simulink model "AGC30Model_ex1_11"  (R2021a)
settings: Solver=ode4  StartTime=stime  StopTime=etime  FixedStep=dtload  RelTol=1e-3
values from neighbouring files (symbols this model uses):
  AL_A = 0.3    [init_lfc_model.m]
  AL_B = 0.3    [init_lfc_model.m]
  DELTA_CC = Delta_cc_ty(TY_CC)    [load_thermal_constants.m]
  DELTA_ST = Delta_st_ty(TY_ST)    [load_thermal_constants.m]
  dtload = 0.1    [initset_dataload.m]
  F0 = 60    [init_inertia_model.m]    (also in initset_inertia.m)
  FFCS0_CC = (WF0_CC-WF_MIN_CC)./(1.0-WF_MIN_CC)    [calc_thermal_init_values.m]    (also in init_thermals.m)
  FGT_CC = Fgt_cc_ty(TY_CC)    [load_thermal_constants.m]
  FX_FB_CC = Fx_fb_cc_ty(:,TY_CC)    [load_thermal_constants.m]
  FX_FB_ST = Fx_fb_st_ty(:,TY_ST)    [load_thermal_constants.m]
  FX_FB_WT = FX_FB_WT_ty(:,TY_WT)    [load_const_hydro_constants.m]
  FX_N_GN_VA = FX_N_GN_VA_ty(:,TY_VA)    [load_var_hydro_constants.m]
  FX_N_PM_VA = FX_N_PM_VA_ty(:,TY_VA)    [load_var_hydro_constants.m]
  FX_PTHD_ST = Fx_pthd_st_ty(:,TY_ST)    [load_thermal_constants.m]
  FX_T_PM_VA = FX_T_PM_VA_ty(:,TY_VA)    [load_var_hydro_constants.m]
  FX_TE1_CC = Fx_te1_cc_ty(:,TY_CC)    [load_thermal_constants.m]
  FX_TE2_CC = Fx_te2_cc_ty(:,TY_CC)    [load_thermal_constants.m]
  FX_Y_GN_VA = FX_Y_GN_VA_ty(:,TY_VA)    [load_var_hydro_constants.m]
  FX_Y_PM_VA = FX_Y_PM_VA_ty(:,TY_VA)    [load_var_hydro_constants.m]
  FY_FB_CC = Fy_fb_cc_ty(:,TY_CC)    [load_thermal_constants.m]
  FY_FB_ST = Fy_fb_st_ty(:,TY_ST)    [load_thermal_constants.m]
  FY_FB_WT = FY_FB_WT_ty(:,TY_WT)    [load_const_hydro_constants.m]
  FY_N_GN_VA = FY_N_GN_VA_ty(:,TY_VA)    [load_var_hydro_constants.m]
  FY_N_PM_VA = FY_N_PM_VA_ty(:,TY_VA)    [load_var_hydro_constants.m]
  FY_PTHD_ST = Fy_pthd_st_ty(:,TY_ST)    [load_thermal_constants.m]
  FY_T_PM_VA = FY_T_PM_VA_ty(:,TY_VA)    [load_var_hydro_constants.m]
  FY_TE1_CC = Fy_te1_cc_ty(:,TY_CC)    [load_thermal_constants.m]
  FY_TE2_CC = Fy_te2_cc_ty(:,TY_CC)    [load_thermal_constants.m]
  FY_Y_GN_VA = FY_Y_GN_VA_ty(:,TY_VA)    [load_var_hydro_constants.m]
  FY_Y_PM_VA = FY_Y_PM_VA_ty(:,TY_VA)    [load_var_hydro_constants.m]
  G_cost = [Cost(:,3) ... (first row only)    [initset_dataload.m]
  G_down_limit = max(G_down_limit, G_out_pre - G_speed*5)    [calc_edc_output.m]    (also in edc.m; initset_dataload.m = csvread('G_down_plan_limit.csv',0,1))
  G_G_ST = G_g_st_ty(TY_ST)    [load_thermal_constants.m]
  G_speed = u(220:249,1)    [calc_edc_output.m]    (also in edc.m; initset_dataload.m = G_speed(:,1))
  GF_CC = [1, 1, 1, 1, 1,            1, 1, 1, 1, 1]    [init_thermal_model.m]
  GF_ST = [1, 1, 1, 1, 1, 1, 1,            1, 1, 1, 1,            1, 1, 1, 1, 1, 1]    [init_thermal_model.m]
  GMW_CC = Gmw_cc_ty(TY_CC)    [load_thermal_constants.m]
  GMW_ST = Gmw_st_ty(TY_ST)    [load_thermal_constants.m]
  GMW_VA = GMW_VA_ty(TY_VA)    [load_var_hydro_constants.m]
  GMW_WT = GMW_WT_ty(TY_WT)    [load_const_hydro_constants.m]
  HC_CC = Hc_cc_ty(TY_CC)    [load_thermal_constants.m]
  HT_CC = Ht_cc_ty(TY_CC)    [load_thermal_constants.m]
  IGV0_CC = WF0_CC    [calc_thermal_init_values.m]    (also in init_thermals.m)
  inertia_input = inertia_input'    [initset_dataload.m]
  K1_CONV_VA = K1_CONV_VA_ty(TY_VA)    [load_var_hydro_constants.m]
  K1_CONV_WT = K1_CONV_WT_ty(TY_WT)    [load_const_hydro_constants.m]
  K2_SERV_VA = K2_SERV_VA_ty(TY_VA)    [load_var_hydro_constants.m]
  K2_SERV_WT = K2_SERV_WT_ty(TY_WT)    [load_const_hydro_constants.m]
  K_A = 0.1    [init_lfc_model.m]
  K_B = 0.1    [init_lfc_model.m]
  K_G_ST = K_g_st_ty(TY_ST)    [load_thermal_constants.m]
  K_IGV_CC = K_igv_cc_ty(TY_CC)    [load_thermal_constants.m]
  K_L = 2.0    (= 2)    [init_inertia_model.m]    (also in initset_inertia.m)
  K_MW_GV_VA = K_MW_GV_VA_ty(TY_VA)    [load_var_hydro_constants.m]
  K_PREF_ST = K_pref_st_ty(TY_ST)    [load_thermal_constants.m]
  K_SD_VA = K_SD_VA_ty(TY_VA)    [load_var_hydro_constants.m]
  K_SD_WT = K_SD_WT_ty(TY_WT)    [load_const_hydro_constants.m]
  K_SEQ_WT = K_SEQ_WT_ty(TY_WT)    [load_const_hydro_constants.m]
  K_TE_CC = K_te_cc_ty(TY_CC)    [load_thermal_constants.m]
  KD_PID_VA = KD_PID_VA_ty(TY_VA)    [load_var_hydro_constants.m]
  KD_PID_WT = KD_PID_WT_ty(TY_WT)    [load_const_hydro_constants.m]
  KD_SG_GN_VA = KD_SG_GN_VA_ty(TY_VA)    [load_var_hydro_constants.m]
  KD_SG_PM_VA = KD_SG_PM_VA_ty(TY_VA)    [load_var_hydro_constants.m]
  KGT_CC = FGT_CC./((TFR_CC-TER_CC)-(TDR_CC-TIR_CC))    [calc_thermal_init_values.m]    (also in init_thermals.m)
  KI_PID_VA = KI_PID_VA_ty(TY_VA)    [load_var_hydro_constants.m]
  KI_PID_WT = KI_PID_WT_ty(TY_WT)    [load_const_hydro_constants.m]
  KI_SG_GN_VA = KI_SG_GN_VA_ty(TY_VA)    [load_var_hydro_constants.m]
  KI_SG_PM_VA = KI_SG_PM_VA_ty(TY_VA)    [load_var_hydro_constants.m]
  KP_A = 1.0    (= 1)    [init_lfc_model.m]
  KP_B = 1.0    (= 1)    [init_lfc_model.m]
  KP_PID_VA = KP_PID_VA_ty(TY_VA)    [load_var_hydro_constants.m]
  KP_PID_WT = KP_PID_WT_ty(TY_WT)    [load_const_hydro_constants.m]
  KP_SG_GN_VA = KP_SG_GN_VA_ty(TY_VA)    [load_var_hydro_constants.m]
  KP_SG_PM_VA = KP_SG_PM_VA_ty(TY_VA)    [load_var_hydro_constants.m]
  KST_CC = (1.0-FGT_CC)./TER_CC    [calc_thermal_init_values.m]    (also in init_thermals.m)
  L_FUEL_CC = L_fuel_cc_ty(TY_CC)    [load_thermal_constants.m]
  L_G_ST = L_g_st_ty(TY_ST)    [load_thermal_constants.m]
  L_IGV_CC = L_igv_cc_ty(TY_CC)    [load_thermal_constants.m]
  L_LL_ST = L_ll_st_ty(TY_ST)    [load_thermal_constants.m]
  L_MWD_CC = L_mwd_cc_ty(TY_CC)    [load_thermal_constants.m]
  L_MWD_GN_VA = L_MWD_GN_VA_ty(TY_VA)    [load_var_hydro_constants.m]
  L_MWD_PM_VA = L_MWD_PM_VA_ty(TY_VA)    [load_var_hydro_constants.m]
  L_MWD_ST = L_mwd_st_ty(TY_ST)    [load_thermal_constants.m]
  L_MWD_WT = L_MWD_WT_ty(TY_WT)    [load_const_hydro_constants.m]
  L_PREF_CC = L_pref_cc_ty(TY_CC)    [load_thermal_constants.m]
  L_PREF_ST = L_pref_st_ty(TY_ST)    [load_thermal_constants.m]
  LFC_cycle = 5.0    (= 5)    [init_lfc_model.m]
  load_input = load_input(:,stime+1:etime+1)    [initset_dataload.m]
  M_VA = M_VA_ty(TY_VA)    [load_var_hydro_constants.m]
  MVABase = 1000    [init_inertia_model.m]    (also in initset_inertia.m)
  MW0_ST = zeros(1,17)    [calc_thermal_init_values.m]    (also in init_thermals.m)
  MW0_WT = zeros(1,2)    [calc_const_hydro_init_values.m]    (also in init_conhydros.m)
  P_G_CONV_WT = P_G_CONV_WT_ty(TY_WT)    [load_const_hydro_constants.m]
  PG_INIT_CC = PMWD_SCHEDULE(1,19:28)'    [calc_thermal_init_values.m]    (also in init_thermals.m)
  PLM_CC = Plm_cc_ty(TY_CC)    [load_thermal_constants.m]
  PLM_ST = Plm_st_ty(TY_ST)    [load_thermal_constants.m]
  PMAX_B = 360.0    (= 360)    [init_lfc_model.m]
  PMIN_B = -360.0    (= -360)    [init_lfc_model.m]
  PMST0_CC = zeros(1, 10)    [calc_thermal_init_values.m]    (also in init_thermals.m)
  PMWD_EDC0 = zeros(1,30)    [init_edc_model.m]    (also in initset_edc.m)
  PMWD_SCHEDULE = u(3:32,1)    [calc_edc_output.m]    (also in edc.m; init_edc_model.m = g_out_input'; initset_edc.m = g_out_input')
  PRC_CC = Prc_cc_ty(TY_CC)    [load_thermal_constants.m]
  PRT_CC = PRC_CC.*(1-EP_CC)    [calc_thermal_init_values.m]    (also in init_thermals.m)
  PTH0_ST = zeros(1,17)    [calc_thermal_init_values.m]    (also in init_thermals.m)
  R_LL_ST = R_ll_st_ty(TY_ST)    [load_thermal_constants.m]
  R_MWD_CC = R_mwd_cc_ty(TY_CC)    [load_thermal_constants.m]
  R_MWD_ST = R_mwd_st_ty(TY_ST)    [load_thermal_constants.m]
  R_PREF_CC = R_pref_cc_ty(TY_CC)    [load_thermal_constants.m]
  RA_A = G_speed'    [init_lfc_model.m]
  RA_B = 96.0    (= 96)    [init_lfc_model.m]
  RATE_GN_VA = RATE_GN_VA_ty(TY_VA)    [load_var_hydro_constants.m]
  RATE_PM_VA = RATE_PM_VA_ty(TY_VA)    [load_var_hydro_constants.m]
  RC_CC = Rc_cc_ty(TY_CC)    [load_thermal_constants.m]
  RT_CC = Rt_cc_ty(TY_CC)    [load_thermal_constants.m]
  SW_T_ST = Sw_t_st_ty(TY_ST)    [load_thermal_constants.m]
  T1_B_ST = T1_b_st_ty(TY_ST)    [load_thermal_constants.m]
  T1_CONV_VA = T1_CONV_VA_ty(TY_VA)    [load_var_hydro_constants.m]
  T1_CONV_WT = T1_CONV_WT_ty(TY_WT)    [load_const_hydro_constants.m]
  T1_G_ST = T1_g_st_ty(TY_ST)    [load_thermal_constants.m]
  T2_B_ST = T2_b_st_ty(TY_ST)    [load_thermal_constants.m]
  ... (+53 more)
undefined symbols (not defined in the file or in its folder): DELTA_B, DiscIntNeverNeededParam, FX_FB_ST_OA, FX_PTHD_ST_OA, FY_FB_ST_OA, FY_PTHD_ST_OA, G_G_ST_OA, K_G_ST_OA, K_PREF_ST_OA, MW0_ST_OA, N_GN_INIT_VA, N_PM_INIT_VA, PLM_B, R_LL_ST_OA, T1_B_ST_OA, T1_G_ST_OA, T2_B_ST_OA, T2_G_ST_OA, T3_B_ST_OA, T4_G_ST_OA, T5_G_ST_OA, T_LL_ST_OA, T_PREF_ST_OA, Y_GN_INIT_VA, Y_PM_INIT_VA
libraries: simulink_extras x87, simulink x42, pid_lib x1
(part 4 of 5)

== system AGC30Model_ex1_11/可変速揚水発電機/可変速揚水/連続出力切替 ==
  モデル : Inport
  運転モード : Inport  Port=2
  MWD : Inport  Port=3
  Add : Sum
  Constant : Constant  Value=0
  Gain : Gain  Gain=-1
  Gain1 : Gain  Gain=-1
  Gain2 : Gain  Gain=-1
  MWD使用時に レートを制限 : Switch  Threshold=1
  MWD使用時はMWD-モデル モデル使用時は0 : Switch  Threshold=1
  MWD使用時はMWD-モデルに追従 モデル使用時はレートでMWD-モデルから0へ変化 （MWD⇒モデル時に不連続打消し分として使用） : simulink/Discontinuities/Rate Limiter Dynamic
  Scope1 : Scope
  Scope2 : Scope
  Subtract : Sum  Inputs=-+
  Switch1 : Switch  Threshold=1
  ∞ : Constant  Value=9999
  モデル使用時に レートを制限 : Switch  Threshold=1
  モデル使用時はモデル-MWD MWD使用時は0 : Switch  Threshold=1
  モデル使用時はモデル-MWDに追従 MWD使用時はレートでモデル-MWDから0に変化 （モデル⇒MWD時に不連続打消し分として使用） : simulink/Discontinuities/Rate Limiter Dynamic
  不連続 打消し分 : Switch  Threshold=1
  不連続分を戻すレート : Constant  Value=0.0001
  出力 : Outport  VectorParamsAs1DForOutWhenUnconnected=off
  wires:
  MWD/1 -> Subtract/2, Switch1/3
  モデル/1 -> Switch1/1, Subtract/1
  Constant/1 -> MWD使用時はMWD-モデル モデル使用時は0/1, モデル使用時はモデル-MWD MWD使用時は0/3
  Subtract/1 -> Gain2/1, MWD使用時はMWD-モデル モデル使用時は0/3
  MWD使用時はMWD-モデル モデル使用時は0/1 -> MWD使用時はMWD-モデルに追従 モデル使用時はレートでMWD-モデルから0へ変化 （MWD⇒モデル時に不連続打消し分として使用）/2
  モデル使用時はモデル-MWD MWD使用時は0/1 -> モデル使用時はモデル-MWDに追従 MWD使用時はレートでモデル-MWDから0に変化 （モデル⇒MWD時に不連続打消し分として使用）/2
  モデル使用時はモデル-MWDに追従 MWD使用時はレートでモデル-MWDから0に変化 （モデル⇒MWD時に不連続打消し分として使用）/1 -> 不連続 打消し分/3
  MWD使用時はMWD-モデルに追従 モデル使用時はレートでMWD-モデルから0へ変化 （MWD⇒モデル時に不連続打消し分として使用）/1 -> 不連続 打消し分/1
  Add/1 -> 出力/1
  不連続分を戻すレート/1 -> モデル使用時に レートを制限/1, MWD使用時に レートを制限/3
  ∞/1 -> モデル使用時に レートを制限/3, MWD使用時に レートを制限/1
  モデル使用時に レートを制限/1 -> MWD使用時はMWD-モデルに追従 モデル使用時はレートでMWD-モデルから0へ変化 （MWD⇒モデル時に不連続打消し分として使用）/1, Gain/1
  MWD使用時に レートを制限/1 -> モデル使用時はモデル-MWDに追従 MWD使用時はレートでモデル-MWDから0に変化 （モデル⇒MWD時に不連続打消し分として使用）/1, Gain1/1
  Gain/1 -> MWD使用時はMWD-モデルに追従 モデル使用時はレートでMWD-モデルから0へ変化 （MWD⇒モデル時に不連続打消し分として使用）/3
  Gain1/1 -> モデル使用時はモデル-MWDに追従 MWD使用時はレートでモデル-MWDから0に変化 （モデル⇒MWD時に不連続打消し分として使用）/3
  Gain2/1 -> モデル使用時はモデル-MWD MWD使用時は0/1
  Switch1/1 -> Scope2/1, Add/1
  不連続 打消し分/1 -> Add/2, Scope1/1
  運転モード/1 -> Switch1/2, MWD使用時はMWD-モデル モデル使用時は0/2, モデル使用時はモデル-MWD MWD使用時は0/2, モデル使用時に レートを制限/2, MWD使用時に レートを制限/2, 不連続 打消し分/2

== system AGC30Model_ex1_11/定速揚水発電プラント/Water1/U=1.2L=1 ==
  Inport : Inport
  Constant : Constant  Value=upper_limit
  Constant1 : Constant  Value=lower_limit
  Constant2 : Constant  Value=0
  Constant3 : Constant  Value=0
  Constant4 : Constant  Value=0
  Integrator : Integrator  InitialCondition=X0
  Logical Operator : Logic
  Logical Operator1 : Logic  Operator=OR
  Logical Operator2 : Logic  Operator=OR
  Relational operator : RelationalOperator  Operator=<=  RndMeth=Nearest  InputSameDT=on
  Relational operator1 : RelationalOperator  RndMeth=Nearest  InputSameDT=on
  Relational operator2 : RelationalOperator  Operator=<=  RndMeth=Nearest  InputSameDT=on
  Relational operator3 : RelationalOperator  RndMeth=Nearest  InputSameDT=on
  Saturation : Saturate  UpperLimit=upper_limit  LowerLimit=lower_limit
  Switch : Switch  Threshold=0.5  SaturateOnIntegerOverflow=on  InputSameDT=on
  Outport : Outport  InitialOutput=0  VectorParamsAs1DForOutWhenUnconnected=off
  wires:
  Saturation/1 -> Outport/1
  Inport/1 -> Switch/1, Relational operator2/1, Relational operator3/1
  Switch/1 -> Integrator/1
  Constant/1 -> Relational operator/2
  Constant1/1 -> Relational operator1/2
  Logical Operator/1 -> Switch/2
  Constant2/1 -> Switch/3
  Relational operator/1 -> Logical Operator1/1
  Relational operator2/1 -> Logical Operator1/2
  Logical Operator1/1 -> Logical Operator/1
  Relational operator1/1 -> Logical Operator2/1
  Relational operator3/1 -> Logical Operator2/2
  Logical Operator2/1 -> Logical Operator/2
  Constant3/1 -> Relational operator2/2
  Constant4/1 -> Relational operator3/2
  Integrator/1 -> Saturation/1, Relational operator1/1, Relational operator/1

== system AGC30Model_ex1_11/定速揚水発電プラント/Water1/U=1L=0 ==
  Inport : Inport
  Constant : Constant  Value=upper_limit
  Constant1 : Constant  Value=lower_limit
  Constant2 : Constant  Value=0
  Constant3 : Constant  Value=0
  Constant4 : Constant  Value=0
  Integrator : Integrator  InitialCondition=X0
  Logical Operator : Logic
  Logical Operator1 : Logic  Operator=OR
  Logical Operator2 : Logic  Operator=OR
  Relational operator : RelationalOperator  Operator=<=  RndMeth=Nearest  InputSameDT=on
  Relational operator1 : RelationalOperator  RndMeth=Nearest  InputSameDT=on
  Relational operator2 : RelationalOperator  Operator=<=  RndMeth=Nearest  InputSameDT=on
  Relational operator3 : RelationalOperator  RndMeth=Nearest  InputSameDT=on
  Saturation : Saturate  UpperLimit=upper_limit  LowerLimit=lower_limit
  Switch : Switch  Threshold=0.5  SaturateOnIntegerOverflow=on  InputSameDT=on
  Outport : Outport  InitialOutput=0  VectorParamsAs1DForOutWhenUnconnected=off
  wires:
  Constant4/1 -> Relational operator3/2
  Constant3/1 -> Relational operator2/2
  Logical Operator2/1 -> Logical Operator/2
  Relational operator3/1 -> Logical Operator2/2
  Relational operator1/1 -> Logical Operator2/1
  Logical Operator1/1 -> Logical Operator/1
  Relational operator2/1 -> Logical Operator1/2
  Relational operator/1 -> Logical Operator1/1
  Constant2/1 -> Switch/3
  Logical Operator/1 -> Switch/2
  Constant1/1 -> Relational operator1/2
  Constant/1 -> Relational operator/2
  Switch/1 -> Integrator/1
  Inport/1 -> Switch/1, Relational operator2/1, Relational operator3/1
  Integrator/1 -> Relational operator1/1, Relational operator/1, Saturation/1
  Saturation/1 -> Outport/1

== system AGC30Model_ex1_11/定速揚水発電プラント/Water1/連続出力切替 ==
  モデル : Inport
  運転モード : Inport  Port=2
  MWD : Inport  Port=3
  Add : Sum
  Constant : Constant  Value=0
  Gain : Gain  Gain=-1
  Gain1 : Gain  Gain=-1
  Gain2 : Gain  Gain=-1
  MWD使用時に レートを制限 : Switch  Threshold=1
  MWD使用時はMWD-モデル モデル使用時は0 : Switch  Threshold=1
  MWD使用時はMWD-モデルに追従 モデル使用時はレートでMWD-モデルから0へ変化 （MWD⇒モデル時に不連続打消し分として使用） : simulink/Discontinuities/Rate Limiter Dynamic
  Subtract : Sum  Inputs=-+
  Switch1 : Switch  Threshold=1
  ∞ : Constant  Value=9999
  モデル使用時に レートを制限 : Switch  Threshold=1
  モデル使用時はモデル-MWD MWD使用時は0 : Switch  Threshold=1
  モデル使用時はモデル-MWDに追従 MWD使用時はレートでモデル-MWDから0に変化 （モデル⇒MWD時に不連続打消し分として使用） : simulink/Discontinuities/Rate Limiter Dynamic
  不連続 打消し分 : Switch  Threshold=1
  不連続分を戻すレート : Constant  Value=0.0001
  出力 : Outport  VectorParamsAs1DForOutWhenUnconnected=off
  wires:
  MWD/1 -> Subtract/2, Switch1/3
  モデル/1 -> Switch1/1, Subtract/1
  Constant/1 -> MWD使用時はMWD-モデル モデル使用時は0/1, モデル使用時はモデル-MWD MWD使用時は0/3
  Subtract/1 -> Gain2/1, MWD使用時はMWD-モデル モデル使用時は0/3
  MWD使用時はMWD-モデル モデル使用時は0/1 -> MWD使用時はMWD-モデルに追従 モデル使用時はレートでMWD-モデルから0へ変化 （MWD⇒モデル時に不連続打消し分として使用）/2
  モデル使用時はモデル-MWD MWD使用時は0/1 -> モデル使用時はモデル-MWDに追従 MWD使用時はレートでモデル-MWDから0に変化 （モデル⇒MWD時に不連続打消し分として使用）/2
  モデル使用時はモデル-MWDに追従 MWD使用時はレートでモデル-MWDから0に変化 （モデル⇒MWD時に不連続打消し分として使用）/1 -> 不連続 打消し分/3
  MWD使用時はMWD-モデルに追従 モデル使用時はレートでMWD-モデルから0へ変化 （MWD⇒モデル時に不連続打消し分として使用）/1 -> 不連続 打消し分/1
  Add/1 -> 出力/1
  不連続分を戻すレート/1 -> モデル使用時に レートを制限/1, MWD使用時に レートを制限/3
  ∞/1 -> モデル使用時に レートを制限/3, MWD使用時に レートを制限/1
  モデル使用時に レートを制限/1 -> MWD使用時はMWD-モデルに追従 モデル使用時はレートでMWD-モデルから0へ変化 （MWD⇒モデル時に不連続打消し分として使用）/1, Gain/1
  MWD使用時に レートを制限/1 -> モデル使用時はモデル-MWDに追従 MWD使用時はレートでモデル-MWDから0に変化 （モデル⇒MWD時に不連続打消し分として使用）/1, Gain1/1
  Gain/1 -> MWD使用時はMWD-モデルに追従 モデル使用時はレートでMWD-モデルから0へ変化 （MWD⇒モデル時に不連続打消し分として使用）/3
  Gain1/1 -> モデル使用時はモデル-MWDに追従 MWD使用時はレートでモデル-MWDから0に変化 （モデル⇒MWD時に不連続打消し分として使用）/3
  Gain2/1 -> モデル使用時はモデル-MWD MWD使用時は0/1
  Switch1/1 -> Add/1
  不連続 打消し分/1 -> Add/2
  運転モード/1 -> Switch1/2, MWD使用時はMWD-モデル モデル使用時は0/2, モデル使用時はモデル-MWD MWD使用時は0/2, モデル使用時に レートを制限/2, MWD使用時に レートを制限/2, 不連続 打消し分/2

== system AGC30Model_ex1_11/定速揚水発電プラント/Water2/U=1.2L=1 ==
  Inport : Inport
  Constant : Constant  Value=upper_limit
  Constant1 : Constant  Value=lower_limit
  Constant2 : Constant  Value=0
  Constant3 : Constant  Value=0
  Constant4 : Constant  Value=0
  Integrator : Integrator  InitialCondition=X0
  Logical Operator : Logic
  Logical Operator1 : Logic  Operator=OR
  Logical Operator2 : Logic  Operator=OR
  Relational operator : RelationalOperator  Operator=<=  RndMeth=Nearest  InputSameDT=on
  Relational operator1 : RelationalOperator  RndMeth=Nearest  InputSameDT=on
  Relational operator2 : RelationalOperator  Operator=<=  RndMeth=Nearest  InputSameDT=on
  Relational operator3 : RelationalOperator  RndMeth=Nearest  InputSameDT=on
  Saturation : Saturate  UpperLimit=upper_limit  LowerLimit=lower_limit
  Switch : Switch  Threshold=0.5  SaturateOnIntegerOverflow=on  InputSameDT=on
  Outport : Outport  InitialOutput=0  VectorParamsAs1DForOutWhenUnconnected=off
  wires:
  Saturation/1 -> Outport/1
  Inport/1 -> Switch/1, Relational operator2/1, Relational operator3/1
  Switch/1 -> Integrator/1
  Constant/1 -> Relational operator/2
  Constant1/1 -> Relational operator1/2
  Logical Operator/1 -> Switch/2
  Constant2/1 -> Switch/3
  Relational operator/1 -> Logical Operator1/1
  Relational operator2/1 -> Logical Operator1/2
  Logical Operator1/1 -> Logical Operator/1
  Relational operator1/1 -> Logical Operator2/1
  Relational operator3/1 -> Logical Operator2/2
  Logical Operator2/1 -> Logical Operator/2
  Constant3/1 -> Relational operator2/2
  Constant4/1 -> Relational operator3/2
  Integrator/1 -> Saturation/1, Relational operator1/1, Relational operator/1

== system AGC30Model_ex1_11/定速揚水発電プラント/Water2/U=1L=0 ==
  Inport : Inport
  Constant : Constant  Value=upper_limit
  Constant1 : Constant  Value=lower_limit
  Constant2 : Constant  Value=0
  Constant3 : Constant  Value=0
  Constant4 : Constant  Value=0
  Integrator : Integrator  InitialCondition=X0
  Logical Operator : Logic
  Logical Operator1 : Logic  Operator=OR
  Logical Operator2 : Logic  Operator=OR
  Relational operator : RelationalOperator  Operator=<=  RndMeth=Nearest  InputSameDT=on
  Relational operator1 : RelationalOperator  RndMeth=Nearest  InputSameDT=on
  Relational operator2 : RelationalOperator  Operator=<=  RndMeth=Nearest  InputSameDT=on
  Relational operator3 : RelationalOperator  RndMeth=Nearest  InputSameDT=on
  Saturation : Saturate  UpperLimit=upper_limit  LowerLimit=lower_limit
  Switch : Switch  Threshold=0.5  SaturateOnIntegerOverflow=on  InputSameDT=on
  Outport : Outport  InitialOutput=0  VectorParamsAs1DForOutWhenUnconnected=off
  wires:
  Constant4/1 -> Relational operator3/2
  Constant3/1 -> Relational operator2/2
  Logical Operator2/1 -> Logical Operator/2
  Relational operator3/1 -> Logical Operator2/2
  Relational operator1/1 -> Logical Operator2/1
  Logical Operator1/1 -> Logical Operator/1
  Relational operator2/1 -> Logical Operator1/2
  Relational operator/1 -> Logical Operator1/1
  Constant2/1 -> Switch/3
  Logical Operator/1 -> Switch/2
  Constant1/1 -> Relational operator1/2
  Constant/1 -> Relational operator/2
  Switch/1 -> Integrator/1
  Inport/1 -> Switch/1, Relational operator2/1, Relational operator3/1
  Integrator/1 -> Relational operator1/1, Relational operator/1, Saturation/1
  Saturation/1 -> Outport/1

== system AGC30Model_ex1_11/定速揚水発電プラント/Water2/連続出力切替 ==
  モデル : Inport
  運転モード : Inport  Port=2
  MWD : Inport  Port=3
  Add : Sum
  Constant : Constant  Value=0
  Gain : Gain  Gain=-1
  Gain1 : Gain  Gain=-1
  Gain2 : Gain  Gain=-1
  MWD使用時に レートを制限 : Switch  Threshold=1
  MWD使用時はMWD-モデル モデル使用時は0 : Switch  Threshold=1
  MWD使用時はMWD-モデルに追従 モデル使用時はレートでMWD-モデルから0へ変化 （MWD⇒モデル時に不連続打消し分として使用） : simulink/Discontinuities/Rate Limiter Dynamic
  Subtract : Sum  Inputs=-+
  Switch1 : Switch  Threshold=1
  ∞ : Constant  Value=9999
  モデル使用時に レートを制限 : Switch  Threshold=1
  モデル使用時はモデル-MWD MWD使用時は0 : Switch  Threshold=1
  モデル使用時はモデル-MWDに追従 MWD使用時はレートでモデル-MWDから0に変化 （モデル⇒MWD時に不連続打消し分として使用） : simulink/Discontinuities/Rate Limiter Dynamic
  不連続 打消し分 : Switch  Threshold=1
  不連続分を戻すレート : Constant  Value=0.0001
  出力 : Outport  VectorParamsAs1DForOutWhenUnconnected=off
  wires:
  MWD/1 -> Subtract/2, Switch1/3
  モデル/1 -> Switch1/1, Subtract/1
  Constant/1 -> MWD使用時はMWD-モデル モデル使用時は0/1, モデル使用時はモデル-MWD MWD使用時は0/3
  Subtract/1 -> Gain2/1, MWD使用時はMWD-モデル モデル使用時は0/3
  MWD使用時はMWD-モデル モデル使用時は0/1 -> MWD使用時はMWD-モデルに追従 モデル使用時はレートでMWD-モデルから0へ変化 （MWD⇒モデル時に不連続打消し分として使用）/2
  モデル使用時はモデル-MWD MWD使用時は0/1 -> モデル使用時はモデル-MWDに追従 MWD使用時はレートでモデル-MWDから0に変化 （モデル⇒MWD時に不連続打消し分として使用）/2
  モデル使用時はモデル-MWDに追従 MWD使用時はレートでモデル-MWDから0に変化 （モデル⇒MWD時に不連続打消し分として使用）/1 -> 不連続 打消し分/3
  MWD使用時はMWD-モデルに追従 モデル使用時はレートでMWD-モデルから0へ変化 （MWD⇒モデル時に不連続打消し分として使用）/1 -> 不連続 打消し分/1
  Add/1 -> 出力/1
  不連続分を戻すレート/1 -> モデル使用時に レートを制限/1, MWD使用時に レートを制限/3
  ∞/1 -> モデル使用時に レートを制限/3, MWD使用時に レートを制限/1
  モデル使用時に レートを制限/1 -> MWD使用時はMWD-モデルに追従 モデル使用時はレートでMWD-モデルから0へ変化 （MWD⇒モデル時に不連続打消し分として使用）/1, Gain/1
  MWD使用時に レートを制限/1 -> モデル使用時はモデル-MWDに追従 MWD使用時はレートでモデル-MWDから0に変化 （モデル⇒MWD時に不連続打消し分として使用）/1, Gain1/1
  Gain/1 -> MWD使用時はMWD-モデルに追従 モデル使用時はレートでMWD-モデルから0へ変化 （MWD⇒モデル時に不連続打消し分として使用）/3
  Gain1/1 -> モデル使用時はモデル-MWDに追従 MWD使用時はレートでモデル-MWDから0に変化 （モデル⇒MWD時に不連続打消し分として使用）/3
  Gain2/1 -> モデル使用時はモデル-MWD MWD使用時は0/1
  Switch1/1 -> Add/1
  不連続 打消し分/1 -> Add/2
  運転モード/1 -> Switch1/2, MWD使用時はMWD-モデル モデル使用時は0/2, モデル使用時はモデル-MWD MWD使用時は0/2, モデル使用時に レートを制限/2, MWD使用時に レートを制限/2, 不連続 打消し分/2

== system AGC30Model_ex1_11/汽力プラント/Coal1/追従回路 ==
  In : Inport
  Subtract2 : Sum  Inputs=+-
  追従回路積分1 : Integrator  InitialCondition=MW0_ST(8)/PTH0_ST(8)+PLM_ST(8)  LimitOutput=on  UpperSaturationLimit=U_LL_ST(8)  LowerSaturationLimit=L_LL_ST(8)
  追従変化率 : Saturate  UpperLimit=R_LL_ST(8)/60  LowerLimit=-R_LL_ST(8)/60
  追従時定数 : Gain  Gain=1/T_LL_ST(8)
  Out : Outport  VectorParamsAs1DForOutWhenUnconnected=off
  wires:
  Subtract2/1 -> 追従時定数/1
  追従時定数/1 -> 追従変化率/1
  追従変化率/1 -> 追従回路積分1/1
  追従回路積分1/1 -> Out/1, Subtract2/2
  In/1 -> Subtract2/1

== system AGC30Model_ex1_11/汽力プラント/Coal1/連続出力切替 ==
  モデル : Inport
  運転モード : Inport  Port=2
  MWD : Inport  Port=3
  Add : Sum
  Constant : Constant  Value=0
  Gain : Gain  Gain=-1
  Gain1 : Gain  Gain=-1
  Gain2 : Gain  Gain=-1
  MWD使用時に レートを制限 : Switch  Threshold=1
  MWD使用時はMWD-モデル モデル使用時は0 : Switch  Threshold=1
  MWD使用時はMWD-モデルに追従 モデル使用時はレートでMWD-モデルから0へ変化 （MWD⇒モデル時に不連続打消し分として使用） : simulink/Discontinuities/Rate Limiter Dynamic
  Subtract : Sum  Inputs=-+
  Switch1 : Switch  Threshold=1
  ∞ : Constant  Value=9999
  モデル使用時に レートを制限 : Switch  Threshold=1
  モデル使用時はモデル-MWD MWD使用時は0 : Switch  Threshold=1
  モデル使用時はモデル-MWDに追従 MWD使用時はレートでモデル-MWDから0に変化 （モデル⇒MWD時に不連続打消し分として使用） : simulink/Discontinuities/Rate Limiter Dynamic
  不連続 打消し分 : Switch  Threshold=1
  不連続分を戻すレート : Constant  Value=0.0001
  出力 : Outport  VectorParamsAs1DForOutWhenUnconnected=off
  wires:
  MWD/1 -> Subtract/2, Switch1/3
  モデル/1 -> Switch1/1, Subtract/1
  Constant/1 -> MWD使用時はMWD-モデル モデル使用時は0/1, モデル使用時はモデル-MWD MWD使用時は0/3
  Subtract/1 -> Gain2/1, MWD使用時はMWD-モデル モデル使用時は0/3
  MWD使用時はMWD-モデル モデル使用時は0/1 -> MWD使用時はMWD-モデルに追従 モデル使用時はレートでMWD-モデルから0へ変化 （MWD⇒モデル時に不連続打消し分として使用）/2
  モデル使用時はモデル-MWD MWD使用時は0/1 -> モデル使用時はモデル-MWDに追従 MWD使用時はレートでモデル-MWDから0に変化 （モデル⇒MWD時に不連続打消し分として使用）/2
  モデル使用時はモデル-MWDに追従 MWD使用時はレートでモデル-MWDから0に変化 （モデル⇒MWD時に不連続打消し分として使用）/1 -> 不連続 打消し分/3
  MWD使用時はMWD-モデルに追従 モデル使用時はレートでMWD-モデルから0へ変化 （MWD⇒モデル時に不連続打消し分として使用）/1 -> 不連続 打消し分/1
  Add/1 -> 出力/1
  不連続分を戻すレート/1 -> モデル使用時に レートを制限/1, MWD使用時に レートを制限/3
  ∞/1 -> モデル使用時に レートを制限/3, MWD使用時に レートを制限/1
  モデル使用時に レートを制限/1 -> MWD使用時はMWD-モデルに追従 モデル使用時はレートでMWD-モデルから0へ変化 （MWD⇒モデル時に不連続打消し分として使用）/1, Gain/1
  MWD使用時に レートを制限/1 -> モデル使用時はモデル-MWDに追従 MWD使用時はレートでモデル-MWDから0に変化 （モデル⇒MWD時に不連続打消し分として使用）/1, Gain1/1
  Gain/1 -> MWD使用時はMWD-モデルに追従 モデル使用時はレートでMWD-モデルから0へ変化 （MWD⇒モデル時に不連続打消し分として使用）/3
  Gain1/1 -> モデル使用時はモデル-MWDに追従 MWD使用時はレートでモデル-MWDから0に変化 （モデル⇒MWD時に不連続打消し分として使用）/3
  Gain2/1 -> モデル使用時はモデル-MWD MWD使用時は0/1
  Switch1/1 -> Add/1
  不連続 打消し分/1 -> Add/2
  運転モード/1 -> Switch1/2, MWD使用時はMWD-モデル モデル使用時は0/2, モデル使用時はモデル-MWD MWD使用時は0/2, モデル使用時に レートを制限/2, MWD使用時に レートを制限/2, 不連続 打消し分/2

== system AGC30Model_ex1_11/汽力プラント/Coal2/追従回路 ==
  In : Inport
  Subtract2 : Sum  Inputs=+-
  追従回路積分1 : Integrator  InitialCondition=MW0_ST(8)/PTH0_ST(8)+PLM_ST(8)  LimitOutput=on  UpperSaturationLimit=U_LL_ST(8)  LowerSaturationLimit=L_LL_ST(8)
  追従変化率 : Saturate  UpperLimit=R_LL_ST(8)/60  LowerLimit=-R_LL_ST(8)/60
  追従時定数 : Gain  Gain=1/T_LL_ST(8)
  Out : Outport  VectorParamsAs1DForOutWhenUnconnected=off
  wires:
  In/1 -> Subtract2/1
  追従回路積分1/1 -> Subtract2/2, Out/1
  追従変化率/1 -> 追従回路積分1/1
  追従時定数/1 -> 追従変化率/1
  Subtract2/1 -> 追従時定数/1

== system AGC30Model_ex1_11/汽力プラント/Coal2/連続出力切替 ==
  モデル : Inport
  運転モード : Inport  Port=2
  MWD : Inport  Port=3
  Add : Sum
  Constant : Constant  Value=0
  Gain : Gain  Gain=-1
  Gain1 : Gain  Gain=-1
  Gain2 : Gain  Gain=-1
  MWD使用時に レートを制限 : Switch  Threshold=1
  MWD使用時はMWD-モデル モデル使用時は0 : Switch  Threshold=1
  MWD使用時はMWD-モデルに追従 モデル使用時はレートでMWD-モデルから0へ変化 （MWD⇒モデル時に不連続打消し分として使用） : simulink/Discontinuities/Rate Limiter Dynamic
  Subtract : Sum  Inputs=-+
  Switch1 : Switch  Threshold=1
  ∞ : Constant  Value=9999
  モデル使用時に レートを制限 : Switch  Threshold=1
  モデル使用時はモデル-MWD MWD使用時は0 : Switch  Threshold=1
  モデル使用時はモデル-MWDに追従 MWD使用時はレートでモデル-MWDから0に変化 （モデル⇒MWD時に不連続打消し分として使用） : simulink/Discontinuities/Rate Limiter Dynamic
  不連続 打消し分 : Switch  Threshold=1
  不連続分を戻すレート : Constant  Value=0.0001
  出力 : Outport  VectorParamsAs1DForOutWhenUnconnected=off
  wires:
  運転モード/1 -> 不連続 打消し分/2, MWD使用時に レートを制限/2, モデル使用時に レートを制限/2, モデル使用時はモデル-MWD MWD使用時は0/2, MWD使用時はMWD-モデル モデル使用時は0/2, Switch1/2
  不連続 打消し分/1 -> Add/2
  Switch1/1 -> Add/1
  Gain2/1 -> モデル使用時はモデル-MWD MWD使用時は0/1
  Gain1/1 -> モデル使用時はモデル-MWDに追従 MWD使用時はレートでモデル-MWDから0に変化 （モデル⇒MWD時に不連続打消し分として使用）/3
  Gain/1 -> MWD使用時はMWD-モデルに追従 モデル使用時はレートでMWD-モデルから0へ変化 （MWD⇒モデル時に不連続打消し分として使用）/3
  MWD使用時に レートを制限/1 -> Gain1/1, モデル使用時はモデル-MWDに追従 MWD使用時はレートでモデル-MWDから0に変化 （モデル⇒MWD時に不連続打消し分として使用）/1
  モデル使用時に レートを制限/1 -> Gain/1, MWD使用時はMWD-モデルに追従 モデル使用時はレートでMWD-モデルから0へ変化 （MWD⇒モデル時に不連続打消し分として使用）/1
  ∞/1 -> MWD使用時に レートを制限/1, モデル使用時に レートを制限/3
  不連続分を戻すレート/1 -> MWD使用時に レートを制限/3, モデル使用時に レートを制限/1
  Add/1 -> 出力/1
  MWD使用時はMWD-モデルに追従 モデル使用時はレートでMWD-モデルから0へ変化 （MWD⇒モデル時に不連続打消し分として使用）/1 -> 不連続 打消し分/1
  モデル使用時はモデル-MWDに追従 MWD使用時はレートでモデル-MWDから0に変化 （モデル⇒MWD時に不連続打消し分として使用）/1 -> 不連続 打消し分/3
  モデル使用時はモデル-MWD MWD使用時は0/1 -> モデル使用時はモデル-MWDに追従 MWD使用時はレートでモデル-MWDから0に変化 （モデル⇒MWD時に不連続打消し分として使用）/2
  MWD使用時はMWD-モデル モデル使用時は0/1 -> MWD使用時はMWD-モデルに追従 モデル使用時はレートでMWD-モデルから0へ変化 （MWD⇒モデル時に不連続打消し分として使用）/2
  Subtract/1 -> MWD使用時はMWD-モデル モデル使用時は0/3, Gain2/1
  Constant/1 -> モデル使用時はモデル-MWD MWD使用時は0/3, MWD使用時はMWD-モデル モデル使用時は0/1
  モデル/1 -> Subtract/1, Switch1/1
  MWD/1 -> Switch1/3, Subtract/2

== system AGC30Model_ex1_11/汽力プラント/Coal3/追従回路 ==
  In : Inport
  Subtract2 : Sum  Inputs=+-
  追従回路積分1 : Integrator  InitialCondition=MW0_ST(8)/PTH0_ST(8)+PLM_ST(8)  LimitOutput=on  UpperSaturationLimit=U_LL_ST(8)  LowerSaturationLimit=L_LL_ST(8)
  追従変化率 : Saturate  UpperLimit=R_LL_ST(8)/60  LowerLimit=-R_LL_ST(8)/60
  追従時定数 : Gain  Gain=1/T_LL_ST(8)
  Out : Outport  VectorParamsAs1DForOutWhenUnconnected=off
  wires:
  Subtract2/1 -> 追従時定数/1
  追従時定数/1 -> 追従変化率/1
  追従変化率/1 -> 追従回路積分1/1
  追従回路積分1/1 -> Out/1, Subtract2/2
  In/1 -> Subtract2/1

== system AGC30Model_ex1_11/汽力プラント/Coal3/連続出力切替 ==
  モデル : Inport
  運転モード : Inport  Port=2
  MWD : Inport  Port=3
  Add : Sum
  Constant : Constant  Value=0
  Gain : Gain  Gain=-1
  Gain1 : Gain  Gain=-1
  Gain2 : Gain  Gain=-1
  MWD使用時に レートを制限 : Switch  Threshold=1
  MWD使用時はMWD-モデル モデル使用時は0 : Switch  Threshold=1
  MWD使用時はMWD-モデルに追従 モデル使用時はレートでMWD-モデルから0へ変化 （MWD⇒モデル時に不連続打消し分として使用） : simulink/Discontinuities/Rate Limiter Dynamic
  Subtract : Sum  Inputs=-+
  Switch1 : Switch  Threshold=1
  ∞ : Constant  Value=9999
  モデル使用時に レートを制限 : Switch  Threshold=1
  モデル使用時はモデル-MWD MWD使用時は0 : Switch  Threshold=1
  モデル使用時はモデル-MWDに追従 MWD使用時はレートでモデル-MWDから0に変化 （モデル⇒MWD時に不連続打消し分として使用） : simulink/Discontinuities/Rate Limiter Dynamic
  不連続 打消し分 : Switch  Threshold=1
  不連続分を戻すレート : Constant  Value=0.0001
  出力 : Outport  VectorParamsAs1DForOutWhenUnconnected=off
  wires:
  MWD/1 -> Subtract/2, Switch1/3
  モデル/1 -> Switch1/1, Subtract/1
  Constant/1 -> MWD使用時はMWD-モデル モデル使用時は0/1, モデル使用時はモデル-MWD MWD使用時は0/3
  Subtract/1 -> Gain2/1, MWD使用時はMWD-モデル モデル使用時は0/3
  MWD使用時はMWD-モデル モデル使用時は0/1 -> MWD使用時はMWD-モデルに追従 モデル使用時はレートでMWD-モデルから0へ変化 （MWD⇒モデル時に不連続打消し分として使用）/2
  モデル使用時はモデル-MWD MWD使用時は0/1 -> モデル使用時はモデル-MWDに追従 MWD使用時はレートでモデル-MWDから0に変化 （モデル⇒MWD時に不連続打消し分として使用）/2
  モデル使用時はモデル-MWDに追従 MWD使用時はレートでモデル-MWDから0に変化 （モデル⇒MWD時に不連続打消し分として使用）/1 -> 不連続 打消し分/3
  MWD使用時はMWD-モデルに追従 モデル使用時はレートでMWD-モデルから0へ変化 （MWD⇒モデル時に不連続打消し分として使用）/1 -> 不連続 打消し分/1
  Add/1 -> 出力/1
  不連続分を戻すレート/1 -> モデル使用時に レートを制限/1, MWD使用時に レートを制限/3
  ∞/1 -> モデル使用時に レートを制限/3, MWD使用時に レートを制限/1
  モデル使用時に レートを制限/1 -> MWD使用時はMWD-モデルに追従 モデル使用時はレートでMWD-モデルから0へ変化 （MWD⇒モデル時に不連続打消し分として使用）/1, Gain/1
  MWD使用時に レートを制限/1 -> モデル使用時はモデル-MWDに追従 MWD使用時はレートでモデル-MWDから0に変化 （モデル⇒MWD時に不連続打消し分として使用）/1, Gain1/1
  Gain/1 -> MWD使用時はMWD-モデルに追従 モデル使用時はレートでMWD-モデルから0へ変化 （MWD⇒モデル時に不連続打消し分として使用）/3
  Gain1/1 -> モデル使用時はモデル-MWDに追従 MWD使用時はレートでモデル-MWDから0に変化 （モデル⇒MWD時に不連続打消し分として使用）/3
  Gain2/1 -> モデル使用時はモデル-MWD MWD使用時は0/1
  Switch1/1 -> Add/1
  不連続 打消し分/1 -> Add/2
  運転モード/1 -> Switch1/2, MWD使用時はMWD-モデル モデル使用時は0/2, モデル使用時はモデル-MWD MWD使用時は0/2, モデル使用時に レートを制限/2, MWD使用時に レートを制限/2, 不連続 打消し分/2

== system AGC30Model_ex1_11/汽力プラント/Coal4/追従回路 ==
  In : Inport
  Subtract2 : Sum  Inputs=+-
  追従回路積分1 : Integrator  InitialCondition=MW0_ST(9)/PTH0_ST(9)+PLM_ST(9)  LimitOutput=on  UpperSaturationLimit=U_LL_ST(9)  LowerSaturationLimit=L_LL_ST(9)
  追従変化率 : Saturate  UpperLimit=R_LL_ST(9)/60  LowerLimit=-R_LL_ST(9)/60
  追従時定数 : Gain  Gain=1/T_LL_ST(9)
  Out : Outport  VectorParamsAs1DForOutWhenUnconnected=off
  wires:
  Subtract2/1 -> 追従時定数/1
  追従時定数/1 -> 追従変化率/1
  追従変化率/1 -> 追従回路積分1/1
  追従回路積分1/1 -> Out/1, Subtract2/2
  In/1 -> Subtract2/1

== system AGC30Model_ex1_11/汽力プラント/Coal4/連続出力切替 ==
  モデル : Inport
  運転モード : Inport  Port=2
  MWD : Inport  Port=3
  Add : Sum
  Constant : Constant  Value=0
  Gain : Gain  Gain=-1
  Gain1 : Gain  Gain=-1
  Gain2 : Gain  Gain=-1
  MWD使用時に レートを制限 : Switch  Threshold=1
  MWD使用時はMWD-モデル モデル使用時は0 : Switch  Threshold=1
  MWD使用時はMWD-モデルに追従 モデル使用時はレートでMWD-モデルから0へ変化 （MWD⇒モデル時に不連続打消し分として使用） : simulink/Discontinuities/Rate Limiter Dynamic
  Subtract : Sum  Inputs=-+
  Switch1 : Switch  Threshold=1
  ∞ : Constant  Value=9999
  モデル使用時に レートを制限 : Switch  Threshold=1
  モデル使用時はモデル-MWD MWD使用時は0 : Switch  Threshold=1
  モデル使用時はモデル-MWDに追従 MWD使用時はレートでモデル-MWDから0に変化 （モデル⇒MWD時に不連続打消し分として使用） : simulink/Discontinuities/Rate Limiter Dynamic
  不連続 打消し分 : Switch  Threshold=1
  不連続分を戻すレート : Constant  Value=0.0001
  出力 : Outport  VectorParamsAs1DForOutWhenUnconnected=off
  wires:
  MWD/1 -> Subtract/2, Switch1/3
  モデル/1 -> Switch1/1, Subtract/1
  Constant/1 -> MWD使用時はMWD-モデル モデル使用時は0/1, モデル使用時はモデル-MWD MWD使用時は0/3
  Subtract/1 -> Gain2/1, MWD使用時はMWD-モデル モデル使用時は0/3
  MWD使用時はMWD-モデル モデル使用時は0/1 -> MWD使用時はMWD-モデルに追従 モデル使用時はレートでMWD-モデルから0へ変化 （MWD⇒モデル時に不連続打消し分として使用）/2
  モデル使用時はモデル-MWD MWD使用時は0/1 -> モデル使用時はモデル-MWDに追従 MWD使用時はレートでモデル-MWDから0に変化 （モデル⇒MWD時に不連続打消し分として使用）/2
  モデル使用時はモデル-MWDに追従 MWD使用時はレートでモデル-MWDから0に変化 （モデル⇒MWD時に不連続打消し分として使用）/1 -> 不連続 打消し分/3
  MWD使用時はMWD-モデルに追従 モデル使用時はレートでMWD-モデルから0へ変化 （MWD⇒モデル時に不連続打消し分として使用）/1 -> 不連続 打消し分/1
  Add/1 -> 出力/1
  不連続分を戻すレート/1 -> モデル使用時に レートを制限/1, MWD使用時に レートを制限/3
  ∞/1 -> モデル使用時に レートを制限/3, MWD使用時に レートを制限/1
  モデル使用時に レートを制限/1 -> MWD使用時はMWD-モデルに追従 モデル使用時はレートでMWD-モデルから0へ変化 （MWD⇒モデル時に不連続打消し分として使用）/1, Gain/1
  MWD使用時に レートを制限/1 -> モデル使用時はモデル-MWDに追従 MWD使用時はレートでモデル-MWDから0に変化 （モデル⇒MWD時に不連続打消し分として使用）/1, Gain1/1
  Gain/1 -> MWD使用時はMWD-モデルに追従 モデル使用時はレートでMWD-モデルから0へ変化 （MWD⇒モデル時に不連続打消し分として使用）/3
  Gain1/1 -> モデル使用時はモデル-MWDに追従 MWD使用時はレートでモデル-MWDから0に変化 （モデル⇒MWD時に不連続打消し分として使用）/3
  Gain2/1 -> モデル使用時はモデル-MWD MWD使用時は0/1
  Switch1/1 -> Add/1
  不連続 打消し分/1 -> Add/2
  運転モード/1 -> Switch1/2, MWD使用時はMWD-モデル モデル使用時は0/2, モデル使用時はモデル-MWD MWD使用時は0/2, モデル使用時に レートを制限/2, MWD使用時に レートを制限/2, 不連続 打消し分/2

== system AGC30Model_ex1_11/汽力プラント/Coal5/追従回路 ==
  In : Inport
  Subtract2 : Sum  Inputs=+-
  追従回路積分1 : Integrator  InitialCondition=MW0_ST(10)/PTH0_ST(10)+PLM_ST(10)  LimitOutput=on  UpperSaturationLimit=U_LL_ST(10)  LowerSaturationLimit=L_LL_ST(10)
  追従変化率 : Saturate  UpperLimit=R_LL_ST(10)/60  LowerLimit=-R_LL_ST(10)/60
  追従時定数 : Gain  Gain=1/T_LL_ST(10)
  Out : Outport  VectorParamsAs1DForOutWhenUnconnected=off
  wires:
  Subtract2/1 -> 追従時定数/1
  追従時定数/1 -> 追従変化率/1
  追従変化率/1 -> 追従回路積分1/1
  追従回路積分1/1 -> Out/1, Subtract2/2
  In/1 -> Subtract2/1

== system AGC30Model_ex1_11/汽力プラント/Coal5/連続出力切替 ==
  モデル : Inport
  運転モード : Inport  Port=2
  MWD : Inport  Port=3
  Add : Sum
  Constant : Constant  Value=0
  Gain : Gain  Gain=-1
  Gain1 : Gain  Gain=-1
  Gain2 : Gain  Gain=-1
  MWD使用時に レートを制限 : Switch  Threshold=1
  MWD使用時はMWD-モデル モデル使用時は0 : Switch  Threshold=1
  MWD使用時はMWD-モデルに追従 モデル使用時はレートでMWD-モデルから0へ変化 （MWD⇒モデル時に不連続打消し分として使用） : simulink/Discontinuities/Rate Limiter Dynamic
  Subtract : Sum  Inputs=-+
  Switch1 : Switch  Threshold=1
  ∞ : Constant  Value=9999
  モデル使用時に レートを制限 : Switch  Threshold=1
  モデル使用時はモデル-MWD MWD使用時は0 : Switch  Threshold=1
  モデル使用時はモデル-MWDに追従 MWD使用時はレートでモデル-MWDから0に変化 （モデル⇒MWD時に不連続打消し分として使用） : simulink/Discontinuities/Rate Limiter Dynamic
  不連続 打消し分 : Switch  Threshold=1
  不連続分を戻すレート : Constant  Value=0.0001
  出力 : Outport  VectorParamsAs1DForOutWhenUnconnected=off
  wires:
  MWD/1 -> Subtract/2, Switch1/3
  モデル/1 -> Switch1/1, Subtract/1
  Constant/1 -> MWD使用時はMWD-モデル モデル使用時は0/1, モデル使用時はモデル-MWD MWD使用時は0/3
  Subtract/1 -> Gain2/1, MWD使用時はMWD-モデル モデル使用時は0/3
  MWD使用時はMWD-モデル モデル使用時は0/1 -> MWD使用時はMWD-モデルに追従 モデル使用時はレートでMWD-モデルから0へ変化 （MWD⇒モデル時に不連続打消し分として使用）/2
  モデル使用時はモデル-MWD MWD使用時は0/1 -> モデル使用時はモデル-MWDに追従 MWD使用時はレートでモデル-MWDから0に変化 （モデル⇒MWD時に不連続打消し分として使用）/2
  モデル使用時はモデル-MWDに追従 MWD使用時はレートでモデル-MWDから0に変化 （モデル⇒MWD時に不連続打消し分として使用）/1 -> 不連続 打消し分/3
  MWD使用時はMWD-モデルに追従 モデル使用時はレートでMWD-モデルから0へ変化 （MWD⇒モデル時に不連続打消し分として使用）/1 -> 不連続 打消し分/1
  Add/1 -> 出力/1
  不連続分を戻すレート/1 -> モデル使用時に レートを制限/1, MWD使用時に レートを制限/3
  ∞/1 -> モデル使用時に レートを制限/3, MWD使用時に レートを制限/1
  モデル使用時に レートを制限/1 -> MWD使用時はMWD-モデルに追従 モデル使用時はレートでMWD-モデルから0へ変化 （MWD⇒モデル時に不連続打消し分として使用）/1, Gain/1
  MWD使用時に レートを制限/1 -> モデル使用時はモデル-MWDに追従 MWD使用時はレートでモデル-MWDから0に変化 （モデル⇒MWD時に不連続打消し分として使用）/1, Gain1/1
  Gain/1 -> MWD使用時はMWD-モデルに追従 モデル使用時はレートでMWD-モデルから0へ変化 （MWD⇒モデル時に不連続打消し分として使用）/3
  Gain1/1 -> モデル使用時はモデル-MWDに追従 MWD使用時はレートでモデル-MWDから0に変化 （モデル⇒MWD時に不連続打消し分として使用）/3
  Gain2/1 -> モデル使用時はモデル-MWD MWD使用時は0/1
  Switch1/1 -> Add/1
  不連続 打消し分/1 -> Add/2
  運転モード/1 -> Switch1/2, MWD使用時はMWD-モデル モデル使用時は0/2, モデル使用時はモデル-MWD MWD使用時は0/2, モデル使用時に レートを制限/2, MWD使用時に レートを制限/2, 不連続 打消し分/2

== system AGC30Model_ex1_11/汽力プラント/Coal6/追従回路 ==
  In : Inport
  Subtract2 : Sum  Inputs=+-
  追従回路積分1 : Integrator  InitialCondition=MW0_ST(11)/PTH0_ST(11)+PLM_ST(11)  LimitOutput=on  UpperSaturationLimit=U_LL_ST(11)  LowerSaturationLimit=L_LL_ST(11)
  追従変化率 : Saturate  UpperLimit=R_LL_ST(11)/60  LowerLimit=-R_LL_ST(11)/60
  追従時定数 : Gain  Gain=1/T_LL_ST(11)
  Out : Outport  VectorParamsAs1DForOutWhenUnconnected=off
  wires:
  Subtract2/1 -> 追従時定数/1
  追従時定数/1 -> 追従変化率/1
  追従変化率/1 -> 追従回路積分1/1
  追従回路積分1/1 -> Out/1, Subtract2/2
  In/1 -> Subtract2/1

== system AGC30Model_ex1_11/汽力プラント/Coal6/連続出力切替 ==
  モデル : Inport
  運転モード : Inport  Port=2
  MWD : Inport  Port=3
  Add : Sum
  Constant : Constant  Value=0
  Gain : Gain  Gain=-1
  Gain1 : Gain  Gain=-1
  Gain2 : Gain  Gain=-1
  MWD使用時に レートを制限 : Switch  Threshold=1
  MWD使用時はMWD-モデル モデル使用時は0 : Switch  Threshold=1
  MWD使用時はMWD-モデルに追従 モデル使用時はレートでMWD-モデルから0へ変化 （MWD⇒モデル時に不連続打消し分として使用） : simulink/Discontinuities/Rate Limiter Dynamic
  Subtract : Sum  Inputs=-+
  Switch1 : Switch  Threshold=1
  ∞ : Constant  Value=9999
  モデル使用時に レートを制限 : Switch  Threshold=1
  モデル使用時はモデル-MWD MWD使用時は0 : Switch  Threshold=1
  モデル使用時はモデル-MWDに追従 MWD使用時はレートでモデル-MWDから0に変化 （モデル⇒MWD時に不連続打消し分として使用） : simulink/Discontinuities/Rate Limiter Dynamic
  不連続 打消し分 : Switch  Threshold=1
  不連続分を戻すレート : Constant  Value=0.0001
  出力 : Outport  VectorParamsAs1DForOutWhenUnconnected=off
  wires:
  MWD/1 -> Subtract/2, Switch1/3
  モデル/1 -> Switch1/1, Subtract/1
  Constant/1 -> MWD使用時はMWD-モデル モデル使用時は0/1, モデル使用時はモデル-MWD MWD使用時は0/3
  Subtract/1 -> Gain2/1, MWD使用時はMWD-モデル モデル使用時は0/3
  MWD使用時はMWD-モデル モデル使用時は0/1 -> MWD使用時はMWD-モデルに追従 モデル使用時はレートでMWD-モデルから0へ変化 （MWD⇒モデル時に不連続打消し分として使用）/2
  モデル使用時はモデル-MWD MWD使用時は0/1 -> モデル使用時はモデル-MWDに追従 MWD使用時はレートでモデル-MWDから0に変化 （モデル⇒MWD時に不連続打消し分として使用）/2
  モデル使用時はモデル-MWDに追従 MWD使用時はレートでモデル-MWDから0に変化 （モデル⇒MWD時に不連続打消し分として使用）/1 -> 不連続 打消し分/3
  MWD使用時はMWD-モデルに追従 モデル使用時はレートでMWD-モデルから0へ変化 （MWD⇒モデル時に不連続打消し分として使用）/1 -> 不連続 打消し分/1
  Add/1 -> 出力/1
  不連続分を戻すレート/1 -> モデル使用時に レートを制限/1, MWD使用時に レートを制限/3
  ∞/1 -> モデル使用時に レートを制限/3, MWD使用時に レートを制限/1
  モデル使用時に レートを制限/1 -> MWD使用時はMWD-モデルに追従 モデル使用時はレートでMWD-モデルから0へ変化 （MWD⇒モデル時に不連続打消し分として使用）/1, Gain/1
  MWD使用時に レートを制限/1 -> モデル使用時はモデル-MWDに追従 MWD使用時はレートでモデル-MWDから0に変化 （モデル⇒MWD時に不連続打消し分として使用）/1, Gain1/1
  Gain/1 -> MWD使用時はMWD-モデルに追従 モデル使用時はレートでMWD-モデルから0へ変化 （MWD⇒モデル時に不連続打消し分として使用）/3
  Gain1/1 -> モデル使用時はモデル-MWDに追従 MWD使用時はレートでモデル-MWDから0に変化 （モデル⇒MWD時に不連続打消し分として使用）/3
  Gain2/1 -> モデル使用時はモデル-MWD MWD使用時は0/1
  Switch1/1 -> Add/1
  不連続 打消し分/1 -> Add/2
  運転モード/1 -> Switch1/2, MWD使用時はMWD-モデル モデル使用時は0/2, モデル使用時はモデル-MWD MWD使用時は0/2, モデル使用時に レートを制限/2, MWD使用時に レートを制限/2, 不連続 打消し分/2

== system AGC30Model_ex1_11/汽力プラント/Oil1/追従回路 ==
  In : Inport
  Subtract2 : Sum  Inputs=+-
  追従回路積分 : Integrator  InitialCondition=MW0_ST(1)/PTH0_ST(1)+PLM_ST(1)  LimitOutput=on  UpperSaturationLimit=U_LL_ST(1)  LowerSaturationLimit=L_LL_ST(1)
  追従変化率 : Saturate  UpperLimit=R_LL_ST(1)/60  LowerLimit=-R_LL_ST(1)/60
  追従時定数 : Gain  Gain=1/T_LL_ST(1)
  Out : Outport  VectorParamsAs1DForOutWhenUnconnected=off
  wires:
  Subtract2/1 -> 追従時定数/1
  追従時定数/1 -> 追従変化率/1
  追従変化率/1 -> 追従回路積分/1
  追従回路積分/1 -> Out/1, Subtract2/2
  In/1 -> Subtract2/1

== system AGC30Model_ex1_11/汽力プラント/Oil1/連続出力切替 ==
  モデル : Inport
  運転モード : Inport  Port=2
  MWD : Inport  Port=3
  Add : Sum
  Constant : Constant  Value=0
  Gain : Gain  Gain=-1
  Gain1 : Gain  Gain=-1
  Gain2 : Gain  Gain=-1
  MWD使用時に レートを制限 : Switch  Threshold=1
  MWD使用時はMWD-モデル モデル使用時は0 : Switch  Threshold=1
  MWD使用時はMWD-モデルに追従 モデル使用時はレートでMWD-モデルから0へ変化 （MWD⇒モデル時に不連続打消し分として使用） : simulink/Discontinuities/Rate Limiter Dynamic
  Subtract : Sum  Inputs=-+
  Switch1 : Switch  Threshold=1
  ∞ : Constant  Value=9999
  モデル使用時に レートを制限 : Switch  Threshold=1
  モデル使用時はモデル-MWD MWD使用時は0 : Switch  Threshold=1
  モデル使用時はモデル-MWDに追従 MWD使用時はレートでモデル-MWDから0に変化 （モデル⇒MWD時に不連続打消し分として使用） : simulink/Discontinuities/Rate Limiter Dynamic
  不連続 打消し分 : Switch  Threshold=1
  不連続分を戻すレート : Constant  Value=0.0001
  出力 : Outport  VectorParamsAs1DForOutWhenUnconnected=off
  wires:
  MWD/1 -> Subtract/2, Switch1/3
  モデル/1 -> Switch1/1, Subtract/1
  Constant/1 -> MWD使用時はMWD-モデル モデル使用時は0/1, モデル使用時はモデル-MWD MWD使用時は0/3
  Subtract/1 -> Gain2/1, MWD使用時はMWD-モデル モデル使用時は0/3
  MWD使用時はMWD-モデル モデル使用時は0/1 -> MWD使用時はMWD-モデルに追従 モデル使用時はレートでMWD-モデルから0へ変化 （MWD⇒モデル時に不連続打消し分として使用）/2
  モデル使用時はモデル-MWD MWD使用時は0/1 -> モデル使用時はモデル-MWDに追従 MWD使用時はレートでモデル-MWDから0に変化 （モデル⇒MWD時に不連続打消し分として使用）/2
  モデル使用時はモデル-MWDに追従 MWD使用時はレートでモデル-MWDから0に変化 （モデル⇒MWD時に不連続打消し分として使用）/1 -> 不連続 打消し分/3
  MWD使用時はMWD-モデルに追従 モデル使用時はレートでMWD-モデルから0へ変化 （MWD⇒モデル時に不連続打消し分として使用）/1 -> 不連続 打消し分/1
  Add/1 -> 出力/1
  不連続分を戻すレート/1 -> モデル使用時に レートを制限/1, MWD使用時に レートを制限/3
  ∞/1 -> モデル使用時に レートを制限/3, MWD使用時に レートを制限/1
  モデル使用時に レートを制限/1 -> MWD使用時はMWD-モデルに追従 モデル使用時はレートでMWD-モデルから0へ変化 （MWD⇒モデル時に不連続打消し分として使用）/1, Gain/1
  MWD使用時に レートを制限/1 -> モデル使用時はモデル-MWDに追従 MWD使用時はレートでモデル-MWDから0に変化 （モデル⇒MWD時に不連続打消し分として使用）/1, Gain1/1
  Gain/1 -> MWD使用時はMWD-モデルに追従 モデル使用時はレートでMWD-モデルから0へ変化 （MWD⇒モデル時に不連続打消し分として使用）/3
  Gain1/1 -> モデル使用時はモデル-MWDに追従 MWD使用時はレートでモデル-MWDから0に変化 （モデル⇒MWD時に不連続打消し分として使用）/3
  Gain2/1 -> モデル使用時はモデル-MWD MWD使用時は0/1
  Switch1/1 -> Add/1
  不連続 打消し分/1 -> Add/2
  運転モード/1 -> Switch1/2, MWD使用時はMWD-モデル モデル使用時は0/2, モデル使用時はモデル-MWD MWD使用時は0/2, モデル使用時に レートを制限/2, MWD使用時に レートを制限/2, 不連続 打消し分/2

== system AGC30Model_ex1_11/汽力プラント/Oil2/追従回路 ==
  In : Inport
  Subtract2 : Sum  Inputs=+-
  追従回路積分 : Integrator  InitialCondition=MW0_ST(2)/PTH0_ST(2)+PLM_ST(2)  LimitOutput=on  UpperSaturationLimit=U_LL_ST(2)  LowerSaturationLimit=L_LL_ST(2)
  追従変化率 : Saturate  UpperLimit=R_LL_ST(2)/60  LowerLimit=-R_LL_ST(2)/60
  追従時定数 : Gain  Gain=1/T_LL_ST(2)
  Out : Outport  VectorParamsAs1DForOutWhenUnconnected=off
  wires:
  Subtract2/1 -> 追従時定数/1
  追従時定数/1 -> 追従変化率/1
  追従変化率/1 -> 追従回路積分/1
  追従回路積分/1 -> Out/1, Subtract2/2
  In/1 -> Subtract2/1

== system AGC30Model_ex1_11/汽力プラント/Oil2/連続出力切替 ==
  モデル : Inport
  運転モード : Inport  Port=2
  MWD : Inport  Port=3
  Add : Sum
  Constant : Constant  Value=0
  Gain : Gain  Gain=-1
  Gain1 : Gain  Gain=-1
  Gain2 : Gain  Gain=-1
  MWD使用時に レートを制限 : Switch  Threshold=1
  MWD使用時はMWD-モデル モデル使用時は0 : Switch  Threshold=1
  MWD使用時はMWD-モデルに追従 モデル使用時はレートでMWD-モデルから0へ変化 （MWD⇒モデル時に不連続打消し分として使用） : simulink/Discontinuities/Rate Limiter Dynamic
  Subtract : Sum  Inputs=-+
  Switch1 : Switch  Threshold=1
  ∞ : Constant  Value=9999
  モデル使用時に レートを制限 : Switch  Threshold=1
  モデル使用時はモデル-MWD MWD使用時は0 : Switch  Threshold=1
  モデル使用時はモデル-MWDに追従 MWD使用時はレートでモデル-MWDから0に変化 （モデル⇒MWD時に不連続打消し分として使用） : simulink/Discontinuities/Rate Limiter Dynamic
  不連続 打消し分 : Switch  Threshold=1
  不連続分を戻すレート : Constant  Value=0.0001
  出力 : Outport  VectorParamsAs1DForOutWhenUnconnected=off
  wires:
  MWD/1 -> Subtract/2, Switch1/3
  モデル/1 -> Switch1/1, Subtract/1
  Constant/1 -> MWD使用時はMWD-モデル モデル使用時は0/1, モデル使用時はモデル-MWD MWD使用時は0/3
  Subtract/1 -> Gain2/1, MWD使用時はMWD-モデル モデル使用時は0/3
  MWD使用時はMWD-モデル モデル使用時は0/1 -> MWD使用時はMWD-モデルに追従 モデル使用時はレートでMWD-モデルから0へ変化 （MWD⇒モデル時に不連続打消し分として使用）/2
  モデル使用時はモデル-MWD MWD使用時は0/1 -> モデル使用時はモデル-MWDに追従 MWD使用時はレートでモデル-MWDから0に変化 （モデル⇒MWD時に不連続打消し分として使用）/2
  モデル使用時はモデル-MWDに追従 MWD使用時はレートでモデル-MWDから0に変化 （モデル⇒MWD時に不連続打消し分として使用）/1 -> 不連続 打消し分/3
  MWD使用時はMWD-モデルに追従 モデル使用時はレートでMWD-モデルから0へ変化 （MWD⇒モデル時に不連続打消し分として使用）/1 -> 不連続 打消し分/1
  Add/1 -> 出力/1
  不連続分を戻すレート/1 -> モデル使用時に レートを制限/1, MWD使用時に レートを制限/3
  ∞/1 -> モデル使用時に レートを制限/3, MWD使用時に レートを制限/1
  モデル使用時に レートを制限/1 -> MWD使用時はMWD-モデルに追従 モデル使用時はレートでMWD-モデルから0へ変化 （MWD⇒モデル時に不連続打消し分として使用）/1, Gain/1
  MWD使用時に レートを制限/1 -> モデル使用時はモデル-MWDに追従 MWD使用時はレートでモデル-MWDから0に変化 （モデル⇒MWD時に不連続打消し分として使用）/1, Gain1/1
  Gain/1 -> MWD使用時はMWD-モデルに追従 モデル使用時はレートでMWD-モデルから0へ変化 （MWD⇒モデル時に不連続打消し分として使用）/3
  Gain1/1 -> モデル使用時はモデル-MWDに追従 MWD使用時はレートでモデル-MWDから0に変化 （モデル⇒MWD時に不連続打消し分として使用）/3
  Gain2/1 -> モデル使用時はモデル-MWD MWD使用時は0/1
  Switch1/1 -> Add/1
  不連続 打消し分/1 -> Add/2
  運転モード/1 -> Switch1/2, MWD使用時はMWD-モデル モデル使用時は0/2, モデル使用時はモデル-MWD MWD使用時は0/2, モデル使用時に レートを制限/2, MWD使用時に レートを制限/2, 不連続 打消し分/2

== system AGC30Model_ex1_11/汽力プラント/Oil3/追従回路 ==
  In : Inport
  Subtract2 : Sum  Inputs=+-
  追従回路積分 : Integrator  InitialCondition=MW0_ST(3)/PTH0_ST(3)+PLM_ST(3)  UpperSaturationLimit=U_LL_ST(3)  LowerSaturationLimit=L_LL_ST(3)
  追従変化率 : Saturate  UpperLimit=R_LL_ST(3)/60  LowerLimit=-R_LL_ST(3)/60
  追従時定数 : Gain  Gain=1/T_LL_ST(3)
  Out : Outport  VectorParamsAs1DForOutWhenUnconnected=off
  wires:
  Subtract2/1 -> 追従時定数/1
  追従時定数/1 -> 追従変化率/1
  追従変化率/1 -> 追従回路積分/1
  追従回路積分/1 -> Out/1, Subtract2/2
  In/1 -> Subtract2/1

== system AGC30Model_ex1_11/汽力プラント/Oil3/連続出力切替 ==
  モデル : Inport
  運転モード : Inport  Port=2
  MWD : Inport  Port=3
  Add : Sum
  Constant : Constant  Value=0
  Gain : Gain  Gain=-1
  Gain1 : Gain  Gain=-1
  Gain2 : Gain  Gain=-1
  MWD使用時に レートを制限 : Switch  Threshold=1
  MWD使用時はMWD-モデル モデル使用時は0 : Switch  Threshold=1
  MWD使用時はMWD-モデルに追従 モデル使用時はレートでMWD-モデルから0へ変化 （MWD⇒モデル時に不連続打消し分として使用） : simulink/Discontinuities/Rate Limiter Dynamic
  Subtract : Sum  Inputs=-+
  Switch1 : Switch  Threshold=1
  ∞ : Constant  Value=9999
  モデル使用時に レートを制限 : Switch  Threshold=1
  モデル使用時はモデル-MWD MWD使用時は0 : Switch  Threshold=1
  モデル使用時はモデル-MWDに追従 MWD使用時はレートでモデル-MWDから0に変化 （モデル⇒MWD時に不連続打消し分として使用） : simulink/Discontinuities/Rate Limiter Dynamic
  不連続 打消し分 : Switch  Threshold=1
  不連続分を戻すレート : Constant  Value=0.0001
  出力 : Outport  VectorParamsAs1DForOutWhenUnconnected=off
  wires:
  MWD/1 -> Subtract/2, Switch1/3
  モデル/1 -> Switch1/1, Subtract/1
  Constant/1 -> MWD使用時はMWD-モデル モデル使用時は0/1, モデル使用時はモデル-MWD MWD使用時は0/3
  Subtract/1 -> Gain2/1, MWD使用時はMWD-モデル モデル使用時は0/3
  MWD使用時はMWD-モデル モデル使用時は0/1 -> MWD使用時はMWD-モデルに追従 モデル使用時はレートでMWD-モデルから0へ変化 （MWD⇒モデル時に不連続打消し分として使用）/2
  モデル使用時はモデル-MWD MWD使用時は0/1 -> モデル使用時はモデル-MWDに追従 MWD使用時はレートでモデル-MWDから0に変化 （モデル⇒MWD時に不連続打消し分として使用）/2
  モデル使用時はモデル-MWDに追従 MWD使用時はレートでモデル-MWDから0に変化 （モデル⇒MWD時に不連続打消し分として使用）/1 -> 不連続 打消し分/3
  MWD使用時はMWD-モデルに追従 モデル使用時はレートでMWD-モデルから0へ変化 （MWD⇒モデル時に不連続打消し分として使用）/1 -> 不連続 打消し分/1
  Add/1 -> 出力/1
  不連続分を戻すレート/1 -> モデル使用時に レートを制限/1, MWD使用時に レートを制限/3
  ∞/1 -> モデル使用時に レートを制限/3, MWD使用時に レートを制限/1
  モデル使用時に レートを制限/1 -> MWD使用時はMWD-モデルに追従 モデル使用時はレートでMWD-モデルから0へ変化 （MWD⇒モデル時に不連続打消し分として使用）/1, Gain/1
  MWD使用時に レートを制限/1 -> モデル使用時はモデル-MWDに追従 MWD使用時はレートでモデル-MWDから0に変化 （モデル⇒MWD時に不連続打消し分として使用）/1, Gain1/1
  Gain/1 -> MWD使用時はMWD-モデルに追従 モデル使用時はレートでMWD-モデルから0へ変化 （MWD⇒モデル時に不連続打消し分として使用）/3
  Gain1/1 -> モデル使用時はモデル-MWDに追従 MWD使用時はレートでモデル-MWDから0に変化 （モデル⇒MWD時に不連続打消し分として使用）/3
  Gain2/1 -> モデル使用時はモデル-MWD MWD使用時は0/1
  Switch1/1 -> Add/1
  不連続 打消し分/1 -> Add/2
  運転モード/1 -> Switch1/2, MWD使用時はMWD-モデル モデル使用時は0/2, モデル使用時はモデル-MWD MWD使用時は0/2, モデル使用時に レートを制限/2, MWD使用時に レートを制限/2, 不連続 打消し分/2

== system AGC30Model_ex1_11/汽力プラント/Oil4/追従回路 ==
  In : Inport
  Subtract2 : Sum  Inputs=+-
  追従回路積分1 : Integrator  InitialCondition=MW0_ST(4)/PTH0_ST(4)+PLM_ST(4)  LimitOutput=on  UpperSaturationLimit=U_LL_ST(4)  LowerSaturationLimit=L_LL_ST(4)
  追従変化率 : Saturate  UpperLimit=R_LL_ST(4)/60  LowerLimit=-R_LL_ST(4)/60
  追従時定数 : Gain  Gain=1/T_LL_ST(4)
  Out : Outport  VectorParamsAs1DForOutWhenUnconnected=off
  wires:
  Subtract2/1 -> 追従時定数/1
  追従時定数/1 -> 追従変化率/1
  追従変化率/1 -> 追従回路積分1/1
  追従回路積分1/1 -> Out/1, Subtract2/2
  In/1 -> Subtract2/1

== system AGC30Model_ex1_11/汽力プラント/Oil4/連続出力切替 ==
  モデル : Inport
  運転モード : Inport  Port=2
  MWD : Inport  Port=3
  Add : Sum
  Constant : Constant  Value=0
  Gain : Gain  Gain=-1
  Gain1 : Gain  Gain=-1
  Gain2 : Gain  Gain=-1
  MWD使用時に レートを制限 : Switch  Threshold=1
  MWD使用時はMWD-モデル モデル使用時は0 : Switch  Threshold=1
  MWD使用時はMWD-モデルに追従 モデル使用時はレートでMWD-モデルから0へ変化 （MWD⇒モデル時に不連続打消し分として使用） : simulink/Discontinuities/Rate Limiter Dynamic
  Subtract : Sum  Inputs=-+
  Switch1 : Switch  Threshold=1
  ∞ : Constant  Value=9999
  モデル使用時に レートを制限 : Switch  Threshold=1
  モデル使用時はモデル-MWD MWD使用時は0 : Switch  Threshold=1
  モデル使用時はモデル-MWDに追従 MWD使用時はレートでモデル-MWDから0に変化 （モデル⇒MWD時に不連続打消し分として使用） : simulink/Discontinuities/Rate Limiter Dynamic
  不連続 打消し分 : Switch  Threshold=1
  不連続分を戻すレート : Constant  Value=0.0001
  出力 : Outport  VectorParamsAs1DForOutWhenUnconnected=off
  wires:
  MWD/1 -> Subtract/2, Switch1/3
  モデル/1 -> Switch1/1, Subtract/1
  Constant/1 -> MWD使用時はMWD-モデル モデル使用時は0/1, モデル使用時はモデル-MWD MWD使用時は0/3
  Subtract/1 -> Gain2/1, MWD使用時はMWD-モデル モデル使用時は0/3
  MWD使用時はMWD-モデル モデル使用時は0/1 -> MWD使用時はMWD-モデルに追従 モデル使用時はレートでMWD-モデルから0へ変化 （MWD⇒モデル時に不連続打消し分として使用）/2
  モデル使用時はモデル-MWD MWD使用時は0/1 -> モデル使用時はモデル-MWDに追従 MWD使用時はレートでモデル-MWDから0に変化 （モデル⇒MWD時に不連続打消し分として使用）/2
  モデル使用時はモデル-MWDに追従 MWD使用時はレートでモデル-MWDから0に変化 （モデル⇒MWD時に不連続打消し分として使用）/1 -> 不連続 打消し分/3
  MWD使用時はMWD-モデルに追従 モデル使用時はレートでMWD-モデルから0へ変化 （MWD⇒モデル時に不連続打消し分として使用）/1 -> 不連続 打消し分/1
  Add/1 -> 出力/1
  不連続分を戻すレート/1 -> モデル使用時に レートを制限/1, MWD使用時に レートを制限/3
  ∞/1 -> モデル使用時に レートを制限/3, MWD使用時に レートを制限/1
  モデル使用時に レートを制限/1 -> MWD使用時はMWD-モデルに追従 モデル使用時はレートでMWD-モデルから0へ変化 （MWD⇒モデル時に不連続打消し分として使用）/1, Gain/1
  MWD使用時に レートを制限/1 -> モデル使用時はモデル-MWDに追従 MWD使用時はレートでモデル-MWDから0に変化 （モデル⇒MWD時に不連続打消し分として使用）/1, Gain1/1
  Gain/1 -> MWD使用時はMWD-モデルに追従 モデル使用時はレートでMWD-モデルから0へ変化 （MWD⇒モデル時に不連続打消し分として使用）/3
  Gain1/1 -> モデル使用時はモデル-MWDに追従 MWD使用時はレートでモデル-MWDから0に変化 （モデル⇒MWD時に不連続打消し分として使用）/3
  Gain2/1 -> モデル使用時はモデル-MWD MWD使用時は0/1
  Switch1/1 -> Add/1
  不連続 打消し分/1 -> Add/2
  運転モード/1 -> Switch1/2, MWD使用時はMWD-モデル モデル使用時は0/2, モデル使用時はモデル-MWD MWD使用時は0/2, モデル使用時に レートを制限/2, MWD使用時に レートを制限/2, 不連続 打消し分/2

== system AGC30Model_ex1_11/GTCCプラント/GTCC1/ガスタービン/出力特性 ==
  大気温度 : Inport
  圧縮機出口温度 : Inport  Port=2
  ガスタービン入口温度 : Inport  Port=3
  排ガス温度 : Inport  Port=4
  空気流量 : Inport  Port=5
  Add1 : Sum  Inputs=+--+
  Product2 : Product  Inputs=3  RndMeth=Zero
  ガスタービン出力係数 : Constant  Value=KGT_CC(1)
  ガスタービン出力 : Outport  VectorParamsAs1DForOutWhenUnconnected=off
  wires:
  Add1/1 -> Product2/1
  ガスタービン入口温度/1 -> Add1/1
  排ガス温度/1 -> Add1/2
  圧縮機出口温度/1 -> Add1/3
  大気温度/1 -> Add1/4
  空気流量/1 -> Product2/2
  ガスタービン出力係数/1 -> Product2/3
  Product2/1 -> ガスタービン出力/1

== system AGC30Model_ex1_11/GTCCプラント/GTCC1/ガスタービン/温度特性 ==
  燃料流量 : Inport
  空気流量 : Inport  Port=2
  ガスタービン入口温度算出部 : Subsystem
  圧縮機出口温度算出部 : Subsystem
  排ガス温度算出部 : Subsystem
  大気温度 : Outport  VectorParamsAs1DForOutWhenUnconnected=off
  圧縮機出口温度 : Outport  Port=2  VectorParamsAs1DForOutWhenUnconnected=off
  ガスタービン入口温度 : Outport  Port=3  VectorParamsAs1DForOutWhenUnconnected=off
  排ガス温度 : Outport  Port=4  VectorParamsAs1DForOutWhenUnconnected=off
  wires:
  圧縮機出口温度算出部/1(圧縮機出口温度) -> ガスタービン入口温度算出部/3(圧縮機入口温度), 圧縮機出口温度/1
  空気流量/1 -> ガスタービン入口温度算出部/2(空気流量), 圧縮機出口温度算出部/1(空気流量), 排ガス温度算出部/2(空気流量)
  ガスタービン入口温度算出部/1(ガスタービン入口温度) -> ガスタービン入口温度/1, 排ガス温度算出部/1(ガスタービン入口温度)
  排ガス温度算出部/1(排ガス温度) -> 排ガス温度/1
  燃料流量/1 -> ガスタービン入口温度算出部/1(燃料流量)
  圧縮機出口温度算出部/2(大気温度) -> 大気温度/1

== system AGC30Model_ex1_11/GTCCプラント/GTCC1/ガスタービン/空気流量 ==
  IGV開度 : Inport
  周波数偏差 : Inport  Port=2
  Product : Product  Inputs=3
  定格周波数[pu] : Constant
  空気密度比 : Constant  Value=TIR_CC(1)/TI_CC(1)
  系統周波数[pu] : Sum
  空気流量 : Outport  VectorParamsAs1DForOutWhenUnconnected=off
  wires:
  周波数偏差/1 -> 系統周波数[pu]/1
  定格周波数[pu]/1 -> 系統周波数[pu]/2
  空気密度比/1 -> Product/3
  系統周波数[pu]/1 -> Product/2
  IGV開度/1 -> Product/1
  Product/1 -> 空気流量/1

== system AGC30Model_ex1_11/可変速揚水発電機/可変速揚水/揚水運転/励磁装置および発電電動機 ==
  In1 : Inport
  Out1 : Outport  VectorParamsAs1DForOutWhenUnconnected=off
  wires:
  In1/1 -> Out1/1

== system AGC30Model_ex1_11/可変速揚水発電機/可変速揚水/発電運転/励磁装置および発電電動機 ==
  In1 : Inport
  Out1 : Outport  VectorParamsAs1DForOutWhenUnconnected=off
  wires:
  In1/1 -> Out1/1
